simulink model "evolucion_voltaje"  (R2022b)
settings: Solver=VariableStepAuto  StartTime=0.0  StopTime=10.0  RelTol=1e-3
settings Model: Creator=Nacho Andrade  LastModifiedBy=Nacho Andrade

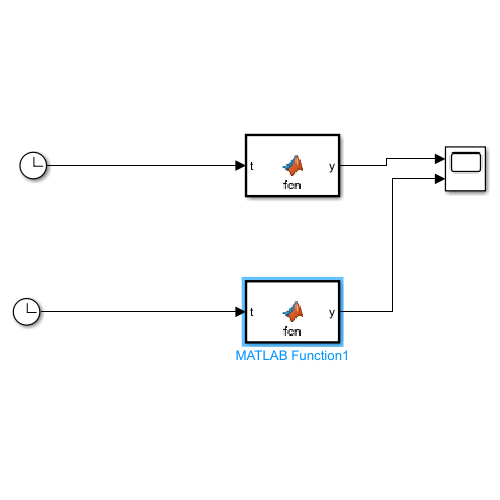
[thumbnail: Simulink's stored preview of the top-level diagram]
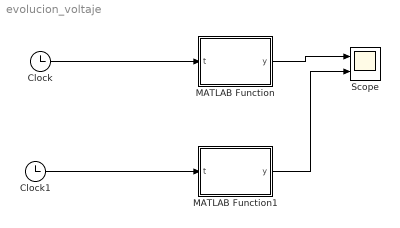
== system evolucion_voltaje ==
  Clock : Clock
  Clock1 : Clock
  MATLAB Function : MATLAB Function  TreatAsAtomicUnit=on
  MATLAB Function1 : MATLAB Function  TreatAsAtomicUnit=on
  Scope : Scope  NumInputPorts=2
  wires:
  Clock/1 -> MATLAB Function/1(t)
  MATLAB Function/1(y) -> Scope/1
  Clock1/1 -> MATLAB Function1/1(t)
  MATLAB Function1/1(y) -> Scope/2

== matlab function evolucion_voltaje/MATLAB Function ==
  data: t input; y output
function y = fcn(t)

y = ((-216*exp(1)/289).*exp(-t))+((216*exp(1)/17).*t.*exp(-t))+((216*exp(1)/289).*exp(-18.*t));

== matlab function evolucion_voltaje/MATLAB Function1 ==
  data: t input; y output
function y = fcn(t)

y = 12.*t.*exp(1-t);
